simulink model "dspcelpcoder"  (Simulink 6.0)
settings: Solver=FixedStepDiscrete  SolverMode=SingleTasking  StartTime=0.0  StopTime=3  RelTol=1e-3
PreLoadFcn:
  | load lpcvocoder.mat;
values from neighbouring files (symbols this model uses):
  D = var(Noisef)    [lmsxy.m]
  Speech = [0.139446526672 0.138625044925 0.138111618832 0.138471017097 0.138316989269 0.138625044925 0.138419674488 0.137854905786 0.138419674488 0.138111618832 0.138573702316 0.138881757971 ... (24000 elements, 24000x1)]    [lpcvocoder.mat]
undefined symbols (not defined in the file or in its folder): jet, magnitude, poly2lsf
libraries: simulink x25, dspindex x17, dspcelplib x14, dsparch4 x12, dspquant2 x10, dspstat3 x10, dspsrcs4 x8, dspbuff3 x8, dspsigops x7, dspmtrx3 x6, dsplp x5, dspobslib x4
(part 2 of 3)

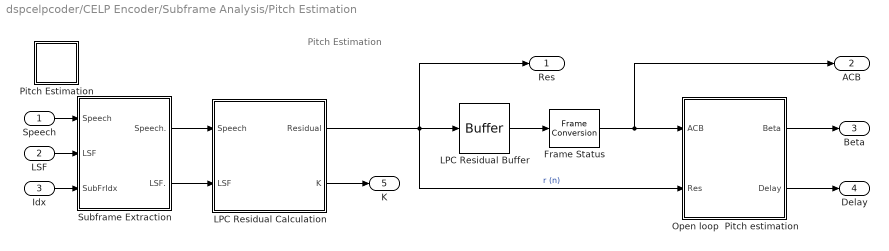
== system dspcelpcoder/CELP Encoder/Subframe Analysis/Pitch Estimation ==
  note: Pitch Estimation
  Speech : Inport  LatchInput=off
  LSF : Inport  Port=2  LatchInput=off
  Idx : Inport  Port=3  LatchInput=off
  Frame Status : FrameConversion  OutFrame=Sample based
  LPC Residual Buffer : dspbuff3/Buffer  N=128+40+20-1  V=187-40  ic=0
  LPC Residual Calculation : Subsystem  PropExecContextAcrossSSBoundary=on
  Open loop  Pitch estimation : Subsystem  PropExecContextAcrossSSBoundary=on
  Pitch Estimation : Subsystem  PropExecContextAcrossSSBoundary=on  mask(DocBlock){ECoderFlag=, DocumentType=Text}
      mask prompts: ECoderFlag "RTW Embedded Coder Flag"; DocumentType "Document Type"
      mask help: Use this block to save long descriptive text with the model. Double-clicking the block will open an editor.
      settings: CopyFcn=docblock('breaklink',gcb);  DeleteFcn=docblock('close_document',gcb);  PreSaveFcn=docblock('save_document',gcb);  OpenFcn=docblock('edit_document',gcb);
      mask StyleString: edit,popup(Text|RTF|HTML)
      mask Display:
      | plot([.8 0 0 1 1 .8 .8 1],[1 1 0 0 .8 1 .8 .8]);
      | text(.5,.5,'DOC','horizontalalignment','center');
  Subframe Extraction : Subsystem  PropExecContextAcrossSSBoundary=on
  Res : Outport
  ACB : Outport  Port=2
  Beta : Outport  Port=3
  Delay : Outport  Port=4
  K : Outport  Port=5
  wires:
  Subframe Extraction/1(Speech.) -> LPC Residual Calculation/1(Speech)
  Subframe Extraction/2(LSF.) -> LPC Residual Calculation/2(LSF)
  LPC Residual Calculation/1(Residual) -> LPC Residual Buffer/1, Open loop  Pitch estimation/2(Res), Res/1  "r (n)"
  LPC Residual Buffer/1 -> Frame Status/1
  Speech/1 -> Subframe Extraction/1(Speech)
  Open loop  Pitch estimation/1(Beta) -> Beta/1
  LSF/1 -> Subframe Extraction/2(LSF)
  LPC Residual Calculation/2(K) -> K/1
  Idx/1 -> Subframe Extraction/3(SubFrIdx)
  Open loop  Pitch estimation/2(Delay) -> Delay/1
  Frame Status/1 -> ACB/1, Open loop  Pitch estimation/1(ACB)

== system dspcelpcoder/CELP Encoder/Subframe Analysis/Pitch Residual computation ==
  note: r (n-D)
  note: beta.r (n-D)
  Res : Inport  LatchInput=off
  ACB : Inport  Port=2  LatchInput=off
  Beta : Inport  Port=3  LatchInput=off
  Delay : Inport  Port=4  LatchInput=off
  Adaptive codebook (ACB) vector candidate  generation : dspcelplib/Select Rows  numRows=40
  DocBlock : Subsystem  PropExecContextAcrossSSBoundary=on  mask(DocBlock){ECoderFlag=, DocumentType=Text}
      mask prompts: ECoderFlag "RTW Embedded Coder Flag"; DocumentType "Document Type"
      mask help: Use this block to save long descriptive text with the model. Double-clicking the block will open an editor.
      settings: CopyFcn=docblock('breaklink',gcb);  DeleteFcn=docblock('close_document',gcb);  PreSaveFcn=docblock('save_document',gcb);  OpenFcn=docblock('edit_document',gcb);
      mask StyleString: edit,popup(Text|RTF|HTML)
      mask Display:
      | plot([.8 0 0 1 1 .8 .8 1],[1 1 0 0 .8 1 .8 .8]);
      | text(.5,.5,'DOC','horizontalalignment','center');
  Frame Status : FrameConversion  OutFrame=Sample based
  Product : Product  SaturateOnIntegerOverflow=on  InputSameDT=on
  SQ (6bits):  Pitch gain (beta) : dspquant2/Scalar Quantizer Encoder  paramSrc=Specify via dialog  partType=Unbounded  BBoundary=[1:10]  UBoundary="[-664.4987     -226.6211     -163.1446     -118.9086     -113.9219     -108.7279     -104.5664     -99.11397     -94.05304     -88.82067     -84.78541     -82.84984      -79.8832     -76.88246     -75.50286     -73.83455     -72.61365     -70.82638      -68.5152     -66.00678     -64.26053     -63.33299     -62.29661     -61.59388     -60.91468      -59.5846     -58.31332     -57.45637     -56.60959     -55.83433     -55.12464     -54.17846     -53.21915     -52.48859     -51.37979     -49.84736     -47.53809     -44.36728     -40.84603     -36.95474     -32.52144     -28.08435     -23.77407     -19.41755     -15.15212     -10.81123      -6.70638     -3.562581     -1.573976    -0.6202197    0.03800587     0.6992125      2.642395      8.360806      18.00463      30.51523      46.10913      64.72121      84.13315       102.069      123.7346      158.1681      206.6721]"  SearchMethod=Binary  tieBreakRule=Choose the lower index  outQU=on  outQError=off  codebook="[-1082.3569     -246.64044     -206.60177     -119.68735     -118.12987     -109.71395     -107.74187     -101.39102     -96.836918     -91.269156     -86.372177     -83.198634     -82.501047     -77.265358     -76.499561     -74.506154     -73.162943     -72.064354     -69.588398     -67.441995     -64.571558     -63.949501     -62.716478     -61.876738     -61.311021     -60.518343     -58.650854     -57.975792     -56.936942     -56.282238     -55.386427     -54.862852     -53.494072      -52.94422     -52.032961      -50.72662     -48.968103      -46.10807       -42.6265     -39.065568     -34.843913     -30.198965     -25.969732     -21.578415     -17.256677     -13.047571     -8.5748944     -4.8378646     -2.2872972    -0.86065481    -0.37978458     0.45579633     0.94262874      4.3421606      12.379451      23.629803       37.40066      54.817595      74.624825      93.641473      110.49643      136.97269      179.36351      233.98073]"  outStatus=off  invalidin=Clip  idtype=int32  roundingMode=Floor  overflowMode=off
  Sum2 : Sum  Inputs=|+-  SaturateOnIntegerOverflow=on
  PitchRes : Outport
  Idx_beta : Outport  Port=2
  wires:
  ACB/1 -> Adaptive codebook (ACB) vector candidate  generation/1
  Sum2/1 -> Frame Status/1
  Res/1 -> Sum2/1  "r(n)"
  Delay/1 -> Adaptive codebook (ACB) vector candidate  generation/2
  Product/1 -> Sum2/2
  Adaptive codebook (ACB) vector candidate  generation/1 -> Product/1
  Beta/1 -> SQ (6bits):  Pitch gain (beta)/1
  SQ (6bits):  Pitch gain (beta)/2 -> Product/2
  SQ (6bits):  Pitch gain (beta)/1 -> Idx_beta/1
  Frame Status/1 -> PitchRes/1

== system dspcelpcoder/CELP Encoder/Subframe Analysis/Subframe Analysis ==
  EmptySubsystem : Subsystem  PropExecContextAcrossSSBoundary=on

== system dspcelpcoder/CELP Decoder/Subframe Synthesis/Formant Post Filter/Subsystem for ARMA Coefficients ==
  Lpc : Inport  LatchInput=off
  Bandwidth Expansion : Subsystem  PropExecContextAcrossSSBoundary=on  mask(Bandwidth Expansion){alpha=0.65}
      mask prompts: alpha "Bandwidth expansion factor:"
      mask help:
      | Generate autoregressive (AR) polynomial with bandwidth expanded relative to the bandwidth of the input AR polynomial.
      |
      | By reducing the radius of the roots in an autoregressive polynomial (i.e., scaling them towards the origin of the Z-plane), the bandwidth of the spectral peaks in the frequency response is expanded (flattened).  This operation is often referred to as "bandwidth expansion".
      |
      | Bandwidth expansion factor must be in the range [0,1], where 1.0 yields no changes to the roots of the polynomial.
      mask Help: web(dspbhelp);
      mask Display: fprintf('Bandwidth\nExpansion\n%g', alpha)
  Bandwidth Expansion1 : Subsystem  PropExecContextAcrossSSBoundary=on  mask(Bandwidth Expansion){alpha=0.75}
      mask prompts: alpha "Bandwidth expansion factor:"
      mask help:
      | Generate autoregressive (AR) polynomial with bandwidth expanded relative to the bandwidth of the input AR polynomial.
      |
      | By reducing the radius of the roots in an autoregressive polynomial (i.e., scaling them towards the origin of the Z-plane), the bandwidth of the spectral peaks in the frequency response is expanded (flattened).  This operation is often referred to as "bandwidth expansion".
      |
      | Bandwidth expansion factor must be in the range [0,1], where 1.0 yields no changes to the roots of the polynomial.
      mask Help: web(dspbhelp);
      mask Display: fprintf('Bandwidth\nExpansion\n%g', alpha)
  FirCoef : Outport
  IirCoef : Outport  Port=2
  wires:
  Lpc/1 -> Bandwidth Expansion/1(In1), Bandwidth Expansion1/1(In1)
  Bandwidth Expansion1/1(Out1) -> IirCoef/1
  Bandwidth Expansion/1(Out1) -> FirCoef/1

== system dspcelpcoder/CELP Decoder/Subframe Synthesis/Gain Scaling Unit/For Iterator Subsystem1 ==
  note: g(n)
  note: y(n)
  note: y(n)=g(n)+0.9375y(n-1)
      | with IC=1
  note: Computation of gain scaling factor for each sample of the subframe
  ScalarGain : Inport  LatchInput=off
  Assignment : Assignment  ElementSrc=External  Rows=-1  ColumnSrc=External
  Constant1 : Constant  Orientation=down  Value=zeros(40,1)  VectorParams1D=off
  For Iterator : ForIterator  IterationLimit=40
  filter : dsparch4/Digital Filter  DialogController=dspDDGCreate  DialogControllerArgs=DataTag8  TypePopup=IIR (all poles)  IIRFiltStruct=Direct form II transposed  AllPoleFiltStruct=Direct form  FIRFiltStruct=Direct form  CoeffSource=Specify via dialog  NumCoeffs=[1 -.95]  DenCoeffs="[1   -0.9375]"  BiQuadCoeffs=[1 0.3 0.4 1 0.1 0.2]  LatticeCoeffs=[0.2 0.4]  denIgnore=on  FiltPerSampPopup=One filter per frame  IC=1  ICnum=0  ICden=0  roundingMode=Floor  overflowMode=off  ScaleValues=1  scaleValueFracLength=14  stageInFracLength=15  stageOutFracLength=15
  VectorGain : Outport
  wires:
  For Iterator/1 -> Assignment/3
  Assignment/1 -> VectorGain/1
  Constant1/1 -> Assignment/1
  ScalarGain/1 -> filter/1
  filter/1 -> Assignment/2

== system dspcelpcoder/CELP Decoder/Subframe Synthesis/Reconstruction of  Speech Subframe/Harmonic Shaper ==
  inRes : Inport  LatchInput=off
  Delay : Inport  Port=2  LatchInput=off
  Beta : Inport  Port=3  LatchInput=off
  1-bz^(-D)2 : Subsystem  TreatAsAtomicUnit=on  PropExecContextAcrossSSBoundary=on
  Energy normalization : Subsystem  PropExecContextAcrossSSBoundary=on
  Pitch Synthesis Filtering 1/(1-b.z^(-D))2 : dsparch4/Digital Filter  DialogController=dspDDGCreate  DialogControllerArgs=DataTag9  TypePopup=IIR (all poles)  IIRFiltStruct=Direct form II transposed  AllPoleFiltStruct=Direct form  FIRFiltStruct=Direct form  CoeffSource=Input port(s)  NumCoeffs=[1 -.95]  DenCoeffs=[1 0.1]  BiQuadCoeffs=[1 0.3 0.4 1 0.1 0.2]  LatticeCoeffs=[0.2 0.4]  denIgnore=on  FiltPerSampPopup=One filter per frame  IC=0  ICnum=0  ICden=0  roundingMode=Floor  overflowMode=off  ScaleValues=1  scaleValueFracLength=14  stageInFracLength=15  stageOutFracLength=15
  OutRes : Outport
  wires:
  Pitch Synthesis Filtering 1/(1-b.z^(-D))2/1 -> Energy normalization/2(SigNew)
  inRes/1 -> Energy normalization/1(SigOrg), Pitch Synthesis Filtering 1/(1-b.z^(-D))2/1
  1-bz^(-D)2/1(Polynom) -> Pitch Synthesis Filtering 1/(1-b.z^(-D))2/2
  Delay/1 -> 1-bz^(-D)2/1(D_buf_1based)
  Beta/1 -> 1-bz^(-D)2/2(beta)
  Energy normalization/1(SigNew2) -> OutRes/1  "res"

== system dspcelpcoder/CELP Decoder/Subframe Synthesis/Reconstruction of  Speech Subframe/LP Synthesis Filter ==
  Residual : Inport  LatchInput=off
  LSF : Inport  Port=2  LatchInput=off
  LPC to/from RC : dsplp/LPC to//from RC  conversion=LPC to RC  perr=off  stability=off  error=Replace it with 1
  LSF/LSP to LPC Conversion : dsplp/LSF//LSP to LPC Conversion  input=LSF in range (0 pi)
  Time-Varying  Synthesis Filter 1/A(z) : dsparch4/Digital Filter  DialogController=dspDDGCreate  DialogControllerArgs=DataTag10  TypePopup=IIR (all poles)  IIRFiltStruct=Direct form II transposed  AllPoleFiltStruct=Lattice AR  FIRFiltStruct=Direct form  CoeffSource=Input port(s)  NumCoeffs=[1 -.95]  DenCoeffs=[1 0.1]  BiQuadCoeffs=[1 0.3 0.4 1 0.1 0.2]  LatticeCoeffs=[0.2 0.4]  denIgnore=off  FiltPerSampPopup=One filter per frame  IC=0  ICnum=0  ICden=0  roundingMode=Floor  overflowMode=off  ScaleValues=1  scaleValueFracLength=14  stageInFracLength=15  stageOutFracLength=15
  Sig : Outport
  LPC : Outport  Port=2
  wires:
  LSF/LSP to LPC Conversion/1 -> LPC to/from RC/1, LPC/1
  LPC to/from RC/1 -> Time-Varying  Synthesis Filter 1/A(z)/2
  Residual/1 -> Time-Varying  Synthesis Filter 1/A(z)/1
  Time-Varying  Synthesis Filter 1/A(z)/1 -> Sig/1  "S(n)"
  LSF/1 -> LSF/LSP to LPC Conversion/1

== system dspcelpcoder/CELP Decoder/Subframe Synthesis/Reconstruction of  Speech Subframe/Pitch synthesis ==
  PitchRes : Inport  LatchInput=off
  Delay : Inport  Port=2  LatchInput=off
  Beta : Inport  Port=3  LatchInput=off
  1-bz^(-D) : Subsystem  TreatAsAtomicUnit=on  PropExecContextAcrossSSBoundary=on
  Pitch synthesis Filter 1/(1-b.z^(-D)) : dsparch4/Digital Filter  DialogController=dspDDGCreate  DialogControllerArgs=DataTag11  TypePopup=IIR (all poles)  IIRFiltStruct=Direct form II transposed  AllPoleFiltStruct=Direct form  FIRFiltStruct=Direct form  CoeffSource=Input port(s)  NumCoeffs=[1 -.95]  DenCoeffs=[1 0.1]  BiQuadCoeffs=[1 0.3 0.4 1 0.1 0.2]  LatticeCoeffs=[0.2 0.4]  denIgnore=on  FiltPerSampPopup=One filter per frame  IC=0  ICnum=0  ICden=0  roundingMode=Floor  overflowMode=off  ScaleValues=1  scaleValueFracLength=14  stageInFracLength=15  stageOutFracLength=15
  LPRes : Outport
  wires:
  1-bz^(-D)/1(Polynom) -> Pitch synthesis Filter 1/(1-b.z^(-D))/2
  Delay/1 -> 1-bz^(-D)/1(D_buf_1based)
  Beta/1 -> 1-bz^(-D)/2(beta)
  PitchRes/1 -> Pitch synthesis Filter 1/(1-b.z^(-D))/1
  Pitch synthesis Filter 1/(1-b.z^(-D))/1 -> LPRes/1

== system dspcelpcoder/CELP Decoder/Subframe Synthesis/Reconstruction of  Speech Subframe/Reconstruction of  Pitch Residual Signal ==
  4SignBit : Inport  LatchInput=off
  4Position : Inport  Port=2  LatchInput=off
  FCBgain : Inport  Port=3  LatchInput=off
  Frame Status : FrameConversion  OutFrame=Sample based
  Frame Status1 : FrameConversion  OutFrame=Sample based
  Product4 : Product  OutDataTypeMode=double  SaturateOnIntegerOverflow=on
  replace 4 selected samples by their sign and set others to zero : Subsystem  TreatAsAtomicUnit=on  PropExecContextAcrossSSBoundary=on
  qPitchRes : Outport
  wires:
  Frame Status/1 -> replace 4 selected samples by their sign and set others to zero/1(4SignBit)
  Frame Status1/1 -> replace 4 selected samples by their sign and set others to zero/2(4Position)
  replace 4 selected samples by their sign and set others to zero/1(newPitchRes) -> Product4/1
  4SignBit/1 -> Frame Status/1
  4Position/1 -> Frame Status1/1
  Product4/1 -> qPitchRes/1
  FCBgain/1 -> Product4/2

== system dspcelpcoder/CELP Encoder/Frame Analysis/Classical LPC analysis/Bandwidth Expansion ==
  In1 : Inport  LatchInput=off
  Window Function : dspsigops/Window Function  DialogController=dspDDGCreate  DialogControllerArgs=DataTag14  winmode=Apply window to input  wintype=User defined  sampmode=Continuous  samptime=1  N=64  Rs=50  beta=10  winsamp=Symmetric  UserWindow=bwexpwin  OptParams=on  UserParams=alpha  dataType=double  isSigned=on  wordLen=16  udDataType=sfix(16)  fracBitsMode=Best precision  numFracBits=15  roundingMode=Floor  overflowMode=off
  Out1 : Outport
  wires:
  In1/1 -> Window Function/1
  Window Function/1 -> Out1/1

== system dspcelpcoder/CELP Encoder/Frame Analysis/Classical LPC analysis/LPC Analysis ==
  EmptySubsystem : Subsystem  PropExecContextAcrossSSBoundary=on

== system dspcelpcoder/CELP Encoder/Frame Analysis/LSF Interpolation/LSF Interpolation ==
  EmptySubsystem : Subsystem  PropExecContextAcrossSSBoundary=on

== system dspcelpcoder/CELP Encoder/Frame Analysis/LSF Vector Quantization/LSF Split VQ ==
  EmptySubsystem : Subsystem  PropExecContextAcrossSSBoundary=on

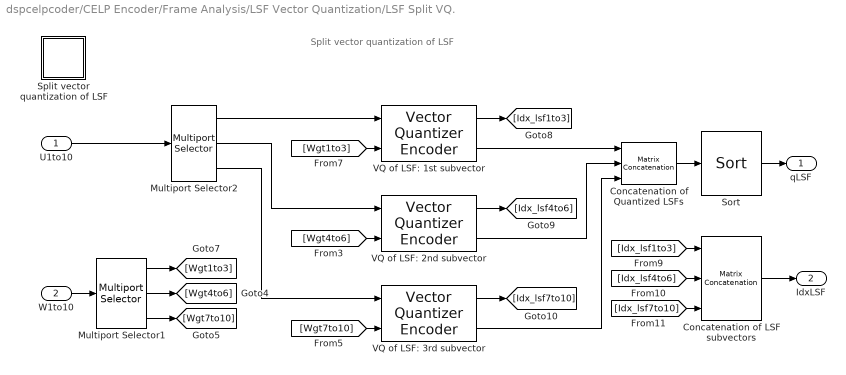
== system dspcelpcoder/CELP Encoder/Frame Analysis/LSF Vector Quantization/LSF Split VQ. ==
  note: Split vector quantization of LSF
  U1to10 : Inport  LatchInput=off
  W1to10 : Inport  Port=2  LatchInput=off
  Concatenation of LSF subvectors : simulink/Math Operations/Matrix Concatenation  numInports=3  catMethod=Horizontal
  Concatenation of Quantized LSFs : simulink/Math Operations/Matrix Concatenation  numInports=3  catMethod=Vertical
  Multiport Selector1 : dspindex/Multiport Selector  rowsOrCols=Rows  idxCellArray={1:3,4:6,7:10}  idxErrMode=Clip Index
  Multiport Selector2 : dspindex/Multiport Selector  rowsOrCols=Rows  idxCellArray={1:3,4:6,7:10}  idxErrMode=Clip Index
  Sort : dspstat3/Sort  DialogController=dspDDGCreate  DialogControllerArgs=DataTag17  otype=Value  dir=Ascending  sortAlg=Quick sort  roundingMode=Floor  overflowMode=off
  Split vector quantization of LSF : Subsystem  PropExecContextAcrossSSBoundary=on  mask(DocBlock){ECoderFlag=, DocumentType=Text}
      mask prompts: ECoderFlag "RTW Embedded Coder Flag"; DocumentType "Document Type"
      mask help: Use this block to save long descriptive text with the model. Double-clicking the block will open an editor.
      settings: CopyFcn=docblock('breaklink',gcb);  DeleteFcn=docblock('close_document',gcb);  PreSaveFcn=docblock('save_document',gcb);  OpenFcn=docblock('edit_document',gcb);
      mask StyleString: edit,popup(Text|RTF|HTML)
      mask Display:
      | plot([.8 0 0 1 1 .8 .8 1],[1 1 0 0 .8 1 .8 .8]);
      | text(.5,.5,'DOC','horizontalalignment','center');
  VQ of LSF: 1st subvector : dspquant2/Vector Quantizer Encoder  CBsource=Specify via dialog  codebook=CB_lsf1to3_10bit  distMeasure=Weighted squared error  wgtSrc=Input port  weights=[1 1 1]  tieBreakRule=Choose the lower index  outQU=on  outQError=off  idtype=int32  roundingMode=Floor  overflowMode=off
  VQ of LSF: 2nd subvector : dspquant2/Vector Quantizer Encoder  CBsource=Specify via dialog  codebook=CB_lsf4to6_10bit  distMeasure=Weighted squared error  wgtSrc=Input port  weights=[1 1 1]  tieBreakRule=Choose the lower index  outQU=on  outQError=off  idtype=int32  roundingMode=Floor  overflowMode=off
  VQ of LSF: 3rd subvector : dspquant2/Vector Quantizer Encoder  CBsource=Specify via dialog  codebook=CB_lsf7to10_10bit  distMeasure=Weighted squared error  wgtSrc=Input port  weights=[1 1 1]  tieBreakRule=Choose the lower index  outQU=on  outQError=off  idtype=int32  roundingMode=Floor  overflowMode=off
  qLSF : Outport
  IdxLSF : Outport  Port=2
  wires:
  VQ of LSF: 1st subvector/2 -> Concatenation of Quantized LSFs/1
  VQ of LSF: 1st subvector/1 -> [Idx_lsf1to3]
  Multiport Selector2/2 -> VQ of LSF: 2nd subvector/1
  Multiport Selector2/3 -> VQ of LSF: 3rd subvector/1
  Multiport Selector1/2 -> [Wgt4to6]
  Multiport Selector1/3 -> [Wgt7to10]
  VQ of LSF: 2nd subvector/1 -> [Idx_lsf4to6]
  [Wgt7to10] -> VQ of LSF: 3rd subvector/2
  VQ of LSF: 3rd subvector/1 -> [Idx_lsf7to10]
  VQ of LSF: 2nd subvector/2 -> Concatenation of Quantized LSFs/2
  Concatenation of Quantized LSFs/1 -> Sort/1
  VQ of LSF: 3rd subvector/2 -> Concatenation of Quantized LSFs/3
  [Wgt4to6] -> VQ of LSF: 2nd subvector/2
  Multiport Selector1/1 -> [Wgt1to3]
  [Wgt1to3] -> VQ of LSF: 1st subvector/2
  [Idx_lsf1to3] -> Concatenation of LSF subvectors/1
  [Idx_lsf4to6] -> Concatenation of LSF subvectors/2
  [Idx_lsf7to10] -> Concatenation of LSF subvectors/3
  W1to10/1 -> Multiport Selector1/1
  U1to10/1 -> Multiport Selector2/1
  Sort/1 -> qLSF/1
  Concatenation of LSF subvectors/1 -> IdxLSF/1
  Multiport Selector2/1 -> VQ of LSF: 1st subvector/1

== system dspcelpcoder/CELP Encoder/Frame Analysis/LSF Vector Quantization/Paliwal Weight  Computation ==
  note: Calculation of Perceptual Weighting Factors
  LSF : Inport  LatchInput=off
  LPC : Inport  Port=2  LatchInput=off
  Calculation of Perceptual  Weighting Factors : Subsystem  PropExecContextAcrossSSBoundary=on  mask(DocBlock){ECoderFlag=, DocumentType=Text}
      mask prompts: ECoderFlag "RTW Embedded Coder Flag"; DocumentType "Document Type"
      mask help: Use this block to save long descriptive text with the model. Double-clicking the block will open an editor.
      settings: CopyFcn=docblock('breaklink',gcb);  DeleteFcn=docblock('close_document',gcb);  PreSaveFcn=docblock('save_document',gcb);  OpenFcn=docblock('edit_document',gcb);
      mask StyleString: edit,popup(Text|RTF|HTML)
      mask Display:
      | plot([.8 0 0 1 1 .8 .8 1],[1 1 0 0 .8 1 .8 .8]);
      | text(.5,.5,'DOC','horizontalalignment','center');
  Constant : Constant  Orientation=up  Value=0.15  VectorParams1D=off  SampleTime=-1
  DSP Gain2 : dspobslib/DSP Gain  gainValue=[ones(1,8) 0.8 0.4]  roundingMode=Floor  overflowMode=off
  DSP Gain3 : dspobslib/DSP Gain  gainValue=-1  roundingMode=Floor  overflowMode=off
  LPCpowSpec : Subsystem  PropExecContextAcrossSSBoundary=on
  Math Function : Math  Operator=pow  SaturateOnIntegerOverflow=on
  Reshape : simulink/Math Operations/Reshape  OutputDimensionality=Column vector  OutputDimensions=[1,1]
  Submatrix : dspmtrx3/Submatrix  RowSpan=Range of rows  RowStartMode=Index  RowStartIndex=2  RowEndMode=Last  RowEndIndex=1  ColSpan=All columns  ColStartMode=First  ColStartIndex=1  ColEndMode=Last  ColEndIndex=1
  Weights : Outport
  wires:
  LPCpowSpec/1(Out) -> Math Function/1
  Constant/1 -> Math Function/2
  Math Function/1 -> DSP Gain2/1
  DSP Gain2/1 -> Reshape/1
  LSF/1 -> LPCpowSpec/2(LSF)
  Reshape/1 -> Weights/1
  Submatrix/1 -> DSP Gain3/1
  LPC/1 -> Submatrix/1
  DSP Gain3/1 -> LPCpowSpec/1(PC)

== system dspcelpcoder/CELP Encoder/Frame Analysis/Subframe Analysis/EmptySubsystem ==

== system dspcelpcoder/CELP Encoder/Subframe Analysis/Innovation signal quantization/DocBlock ==
  EmptySubsystem : Subsystem  PropExecContextAcrossSSBoundary=on

== system dspcelpcoder/CELP Encoder/Subframe Analysis/Innovation signal quantization/Impulse Response ==
  In1 : Inport  LatchInput=off
  DSP Constant : dspsrcs4/DSP Constant  Value=[1;zeros(39,1)]  SampleMode=Discrete  discreteOutput=Frame-based  continuousOutput=Sample-based  sampTime=1  framePeriod=-1  dataType=Inherit from 'Constant value'  isSigned=on  wordLen=16  udDataType=sfix(16)  fracBitsMode=Best precision  numFracBits=15  InterpretAs1D=-inf  Ts=-inf  FramebasedOutput=-inf
  For Iterator Subsystem2 : Subsystem  TreatAsAtomicUnit=on  PropExecContextAcrossSSBoundary=on
      mask Display:
      | disp('Zero State\nIIR Lattice\nFilter');
      | port_label('input',1,'In');
      | port_label('input',2,'K');
      | port_label('output',1,'Out');
  Out1 : Outport
  wires:
  For Iterator Subsystem2/1(SigOut2) -> Out1/1
  In1/1 -> For Iterator Subsystem2/2(K)
  DSP Constant/1 -> For Iterator Subsystem2/1(SigIn2)

== system dspcelpcoder/CELP Encoder/Subframe Analysis/Innovation signal quantization/Searching for FCB pulse  positions and FCB gain ==
  note: To Search for FCB pulse positions and FCB gain
  PitchRes : Inport  LatchInput=off
  Idx : Inport  Port=2  LatchInput=off
  e_n : Inport  Port=3  LatchInput=off
  h : Inport  Port=4  LatchInput=off
  1-based to  0-based : Bias  Bias=-1
  Computation of  Error and Gain : Subsystem  PropExecContextAcrossSSBoundary=on
  For Iterator : ForIterator  ResetStates=reset  IterationLimit=37
  Optimal Features : Subsystem  PropExecContextAcrossSSBoundary=on
  Partial decomposition of  Pitch Residual : Subsystem  PropExecContextAcrossSSBoundary=on
  Searching for FCB features : Subsystem  PropExecContextAcrossSSBoundary=on  mask(DocBlock){ECoderFlag=, DocumentType=Text}
      mask prompts: ECoderFlag "RTW Embedded Coder Flag"; DocumentType "Document Type"
      mask help: Use this block to save long descriptive text with the model. Double-clicking the block will open an editor.
      settings: CopyFcn=docblock('breaklink',gcb);  DeleteFcn=docblock('close_document',gcb);  PreSaveFcn=docblock('save_document',gcb);  OpenFcn=docblock('edit_document',gcb);
      mask StyleString: edit,popup(Text|RTF|HTML)
      mask Display:
      | plot([.8 0 0 1 1 .8 .8 1],[1 1 0 0 .8 1 .8 .8]);
      | text(.5,.5,'DOC','horizontalalignment','center');
  Signal to sign bit : Subsystem  PropExecContextAcrossSSBoundary=on
  pos_sign_g : Outport
  wires:
  1-based to  0-based/1 -> Computation of  Error and Gain/2(4Pos)
  h/1 -> Computation of  Error and Gain/4(h)
  e_n/1 -> Computation of  Error and Gain/3(e_n)
  Signal to sign bit/1(SignBit) -> Computation of  Error and Gain/1(4Val), Optimal Features/1(SignBit)
  Partial decomposition of  Pitch Residual/2(4Idx) -> 1-based to  0-based/1, Optimal Features/4(Pos)
  Partial decomposition of  Pitch Residual/1(4Val) -> Signal to sign bit/1(Sig)
  For Iterator/1 -> Partial decomposition of  Pitch Residual/3(Control)
  Idx/1 -> Partial decomposition of  Pitch Residual/2(Idx)
  PitchRes/1 -> Partial decomposition of  Pitch Residual/1(PitchRes)
  Computation of  Error and Gain/1(Err) -> Optimal Features/2(Err)
  Computation of  Error and Gain/2(G) -> Optimal Features/3(G)
  Optimal Features/1(Features) -> pos_sign_g/1

== system dspcelpcoder/CELP Encoder/Subframe Analysis/Innovation signal quantization/filter ==
  SigIn2 : Inport  LatchInput=off
  K : Inport  Port=2  LatchInput=off
  DocBlock : Subsystem  PropExecContextAcrossSSBoundary=on  mask(DocBlock){ECoderFlag=, DocumentType=Text}
      mask prompts: ECoderFlag "RTW Embedded Coder Flag"; DocumentType "Document Type"
      mask help: Use this block to save long descriptive text with the model. Double-clicking the block will open an editor.
      settings: CopyFcn=docblock('breaklink',gcb);  DeleteFcn=docblock('close_document',gcb);  PreSaveFcn=docblock('save_document',gcb);  OpenFcn=docblock('edit_document',gcb);
      mask StyleString: edit,popup(Text|RTF|HTML)
      mask Display:
      | plot([.8 0 0 1 1 .8 .8 1],[1 1 0 0 .8 1 .8 .8]);
      | text(.5,.5,'DOC','horizontalalignment','center');
  For Iterator : ForIterator  ResetStates=reset  IterationLimit=1  ShowIterationPort=off
  Time-Varying  Synthesis Filter 1/A(z). : dsparch4/Digital Filter  DialogController=dspDDGCreate  DialogControllerArgs=DataTag22  TypePopup=IIR (all poles)  IIRFiltStruct=Direct form II transposed  AllPoleFiltStruct=Lattice AR  FIRFiltStruct=Direct form  CoeffSource=Input port(s)  NumCoeffs=[1 -.95]  DenCoeffs=[1 0.1]  BiQuadCoeffs=[1 0.3 0.4 1 0.1 0.2]  LatticeCoeffs=[0.2 0.4]  denIgnore=off  FiltPerSampPopup=One filter per frame  IC=0  ICnum=0  ICden=0  roundingMode=Floor  overflowMode=off  ScaleValues=1  scaleValueFracLength=14  stageInFracLength=15  stageOutFracLength=15
  SigOut2 : Outport
  wires:
  Time-Varying  Synthesis Filter 1/A(z)./1 -> SigOut2/1
  SigIn2/1 -> Time-Varying  Synthesis Filter 1/A(z)./1
  K/1 -> Time-Varying  Synthesis Filter 1/A(z)./2

== system dspcelpcoder/CELP Encoder/Subframe Analysis/Pitch Estimation/LPC Residual Calculation ==
  Speech : Inport  LatchInput=off
  LSF : Inport  Port=2  LatchInput=off
  LPC to/from RC : dsplp/LPC to//from RC  conversion=LPC to RC  perr=off  stability=off  error=Replace it with 1
  LSF/LSP to LPC Conversion : dsplp/LSF//LSP to LPC Conversion  input=LSF in range (0 pi)
  Time-Varying  Analysis Filter A(z) : dsparch4/Digital Filter  DialogController=dspDDGCreate  DialogControllerArgs=DataTag23  TypePopup=FIR (all zeros)  IIRFiltStruct=Direct form II transposed  AllPoleFiltStruct=Direct form  FIRFiltStruct=Lattice MA  CoeffSource=Input port(s)  NumCoeffs=[1 -.95]  DenCoeffs=[1 0.1]  BiQuadCoeffs=[1 0.3 0.4 1 0.1 0.2]  LatticeCoeffs=[0.2 0.4]  denIgnore=on  FiltPerSampPopup=One filter per frame  IC=0  ICnum=0  ICden=0  roundingMode=Floor  overflowMode=off  ScaleValues=1  scaleValueFracLength=14  stageInFracLength=15  stageOutFracLength=15
  Residual : Outport
  K : Outport  Port=2
  wires:
  LSF/LSP to LPC Conversion/1 -> LPC to/from RC/1
  Speech/1 -> Time-Varying  Analysis Filter A(z)/1
  Time-Varying  Analysis Filter A(z)/1 -> Residual/1
  LSF/1 -> LSF/LSP to LPC Conversion/1
  LPC to/from RC/1 -> Time-Varying  Analysis Filter A(z)/2, K/1

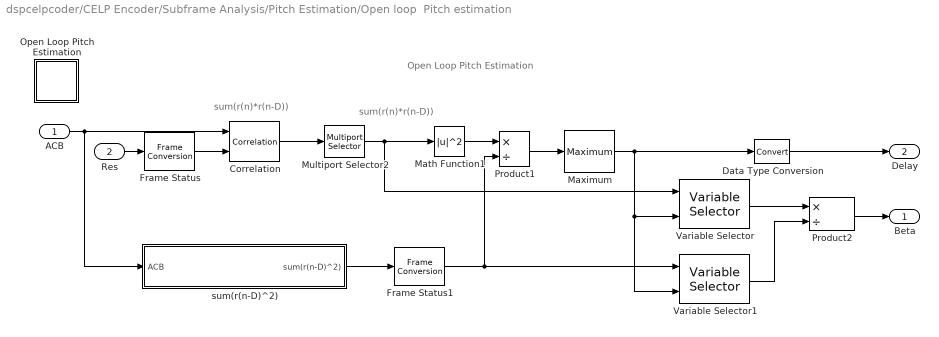
== system dspcelpcoder/CELP Encoder/Subframe Analysis/Pitch Estimation/Open loop  Pitch estimation ==
  note: sum(r(n)*r(n-D))
  note: sum(r(n)*r(n-D))
  note: Open Loop Pitch Estimation
  ACB : Inport  LatchInput=off
  Res : Inport  Port=2  LatchInput=off
  Correlation : dspstat3/Correlation  DialogController=dspDDGCreate  DialogControllerArgs=DataTag24  domain=Fastest  roundingMode=Floor  overflowMode=off
  Data Type Conversion : DataTypeConversion  OutDataTypeMode=int32  SaturateOnIntegerOverflow=on  RndMeth=Zero
  Frame Status : FrameConversion  OutFrame=Sample based
  Frame Status1 : FrameConversion  OutFrame=Sample based
  Math Function1 : Math  Operator=magnitude^2  SaturateOnIntegerOverflow=on
  Maximum : dspstat3/Maximum  DialogController=dspDDGCreate  DialogControllerArgs=DataTag25  fcn=Index  reset=None  roundingMode=Floor  overflowMode=off
  Multiport Selector2 : dspindex/Multiport Selector  rowsOrCols=Rows  idxCellArray={40:167}  idxErrMode=Clip Index
  Open Loop Pitch Estimation : Subsystem  PropExecContextAcrossSSBoundary=on  mask(DocBlock){ECoderFlag=, DocumentType=Text}
      mask prompts: ECoderFlag "RTW Embedded Coder Flag"; DocumentType "Document Type"
      mask help: Use this block to save long descriptive text with the model. Double-clicking the block will open an editor.
      settings: CopyFcn=docblock('breaklink',gcb);  DeleteFcn=docblock('close_document',gcb);  PreSaveFcn=docblock('save_document',gcb);  OpenFcn=docblock('edit_document',gcb);
      mask StyleString: edit,popup(Text|RTF|HTML)
      mask Display:
      | plot([.8 0 0 1 1 .8 .8 1],[1 1 0 0 .8 1 .8 .8]);
      | text(.5,.5,'DOC','horizontalalignment','center');
  Product1 : Product  Inputs=*/  SaturateOnIntegerOverflow=on
  Product2 : Product  Inputs=*/  SaturateOnIntegerOverflow=on
  Variable Selector : dspindex/Variable Selector  rowsOrCols=Rows  IdxMode=Variable  Elements=[1 3]  ZerOneIdxMode=One-based  errmode=Generate Error
  Variable Selector1 : dspindex/Variable Selector  rowsOrCols=Rows  IdxMode=Variable  Elements=[1 3]  ZerOneIdxMode=One-based  errmode=Generate Error
  sum(r(n-D)^2) : Subsystem  TreatAsAtomicUnit=on  PropExecContextAcrossSSBoundary=on
  Beta : Outport
  Delay : Outport  Port=2
  wires:
  Product2/1 -> Beta/1
  Variable Selector/1 -> Product2/1
  Maximum/1 -> Variable Selector1/2, Variable Selector/2, Data Type Conversion/1
  Product1/1 -> Maximum/1
  sum(r(n-D)^2)/1(sum(r(n-D)^2)) -> Frame Status1/1
  Math Function1/1 -> Product1/1
  Res/1 -> Frame Status/1
  ACB/1 -> Correlation/1, sum(r(n-D)^2)/1(ACB)
  Multiport Selector2/1 -> Variable Selector/1, Math Function1/1
  Correlation/1 -> Multiport Selector2/1
  Variable Selector1/1 -> Product2/2
  Frame Status/1 -> Correlation/2
  Frame Status1/1 -> Variable Selector1/1, Product1/2
  Data Type Conversion/1 -> Delay/1

== system dspcelpcoder/CELP Encoder/Subframe Analysis/Pitch Estimation/Pitch Estimation ==
  EmptySubsystem : Subsystem  PropExecContextAcrossSSBoundary=on

== system dspcelpcoder/CELP Encoder/Subframe Analysis/Pitch Estimation/Subframe Extraction ==
  Speech : Inport  LatchInput=off
  LSF : Inport  Port=2  LatchInput=off
  SubFrIdx : Inport  Orientation=up  Port=3  LatchInput=off
  Frame to subframe : simulink/Math Operations/Reshape  OutputDimensionality=Customize  OutputDimensions=[40,4]
  Variable Selector : dspindex/Variable Selector  rowsOrCols=Columns  IdxMode=Variable  Elements=[1 3]  ZerOneIdxMode=One-based  errmode=Generate Error
  Variable Selector2 : dspindex/Variable Selector  rowsOrCols=Columns  IdxMode=Variable  Elements=[1 3]  ZerOneIdxMode=One-based  errmode=Generate Error
  Speech. : Outport
  LSF. : Outport  Port=2
  wires:
  SubFrIdx/1 -> Variable Selector/2, Variable Selector2/2
  Speech/1 -> Frame to subframe/1
  Variable Selector/1 -> Speech./1
  LSF/1 -> Variable Selector2/1
  Variable Selector2/1 -> LSF./1
  Frame to subframe/1 -> Variable Selector/1

== system dspcelpcoder/CELP Encoder/Subframe Analysis/Pitch Residual computation/DocBlock ==
  EmptySubsystem : Subsystem  PropExecContextAcrossSSBoundary=on

== system dspcelpcoder/CELP Encoder/Subframe Analysis/Subframe Analysis/EmptySubsystem ==

== system dspcelpcoder/CELP Decoder/Subframe Synthesis/Formant Post Filter/Subsystem for ARMA Coefficients/Bandwidth Expansion ==
  In1 : Inport  LatchInput=off
  Window Function : dspsigops/Window Function  DialogController=dspDDGCreate  DialogControllerArgs=DataTag4  winmode=Apply window to input  wintype=User defined  sampmode=Continuous  samptime=1  N=64  Rs=50  beta=10  winsamp=Symmetric  UserWindow=bwexpwin  OptParams=on  UserParams=alpha  dataType=double  isSigned=on  wordLen=16  udDataType=sfix(16)  fracBitsMode=Best precision  numFracBits=15  roundingMode=Floor  overflowMode=off
  Out1 : Outport
  wires:
  Window Function/1 -> Out1/1
  In1/1 -> Window Function/1

== system dspcelpcoder/CELP Decoder/Subframe Synthesis/Formant Post Filter/Subsystem for ARMA Coefficients/Bandwidth Expansion1 ==
  In1 : Inport  LatchInput=off
  Window Function : dspsigops/Window Function  DialogController=dspDDGCreate  DialogControllerArgs=DataTag5  winmode=Apply window to input  wintype=User defined  sampmode=Continuous  samptime=1  N=64  Rs=50  beta=10  winsamp=Symmetric  UserWindow=bwexpwin  OptParams=on  UserParams=alpha  dataType=double  isSigned=on  wordLen=16  udDataType=sfix(16)  fracBitsMode=Best precision  numFracBits=15  roundingMode=Floor  overflowMode=off
  Out1 : Outport
  wires:
  In1/1 -> Window Function/1
  Window Function/1 -> Out1/1

== system dspcelpcoder/CELP Decoder/Subframe Synthesis/Reconstruction of  Speech Subframe/Harmonic Shaper/1-bz^(-D)2 ==
  note: 187-40+2 = 149
  D_buf_1based : Inport  LatchInput=off
  beta : Inport  Port=2  LatchInput=off
  Assignment1 : Assignment  ElementSrc=External  Rows=-1  ColumnSrc=External
  DSP Constant : dspsrcs4/DSP Constant  Value=[1 zeros(1,187)]'  SampleMode=Discrete  discreteOutput=Frame-based  continuousOutput=Sample-based  sampTime=1  framePeriod=-1  dataType=double  isSigned=on  wordLen=16  udDataType=sfix(16)  fracBitsMode=Best precision  numFracBits=15  InterpretAs1D=-inf  Ts=-inf  FramebasedOutput=-inf
      settings: additionalParams=on
  DSP Constant1 : dspsrcs4/DSP Constant  Orientation=up  Value=149  SampleMode=Discrete  discreteOutput=Frame-based  continuousOutput=Sample-based  sampTime=-1  framePeriod=-1  dataType=Inherit from 'Constant value'  isSigned=on  wordLen=16  udDataType=sfix(16)  fracBitsMode=Best precision  numFracBits=15  InterpretAs1D=-inf  Ts=-inf  FramebasedOutput=-inf
  DSP Gain : dspobslib/DSP Gain  gainValue=-0.965  roundingMode=Floor  overflowMode=off
  For Iterator : ForIterator  ResetStates=reset  IterationLimit=1  ShowIterationPort=off
  Frame Status1 : FrameConversion  OutFrame=Sample based
  Frame Status2 : FrameConversion  OutFrame=Sample based
  Sum3 : Sum  Inputs=|-+  SaturateOnIntegerOverflow=on
  Polynom : Outport
  wires:
  D_buf_1based/1 -> Sum3/1
  Frame Status2/1 -> Assignment1/3
  DSP Gain/1 -> Assignment1/2
  Sum3/1 -> Frame Status2/1
  DSP Constant1/1 -> Sum3/2
  Frame Status1/1 -> DSP Gain/1
  Assignment1/1 -> Polynom/1
  DSP Constant/1 -> Assignment1/1
  beta/1 -> Frame Status1/1

== system dspcelpcoder/CELP Decoder/Subframe Synthesis/Reconstruction of  Speech Subframe/Harmonic Shaper/Energy normalization ==
  SigOrg : Inport  LatchInput=off
  SigNew : Inport  Port=2  LatchInput=off
  DSP Constant : dspsrcs4/DSP Constant  Orientation=up  Value=eps  SampleMode=Discrete  discreteOutput=Frame-based  continuousOutput=Sample-based  sampTime=1  framePeriod=-1  dataType=Inherit from 'Constant value'  isSigned=on  wordLen=16  udDataType=sfix(16)  fracBitsMode=Best precision  numFracBits=15  InterpretAs1D=-inf  Ts=-inf  FramebasedOutput=-inf
  Math Function1 : Math  Operator=sqrt  SaturateOnIntegerOverflow=on
  Product1 : Product  Inputs=*/  SaturateOnIntegerOverflow=on
  Product2 : Product  SaturateOnIntegerOverflow=on
  Subsystem1 : Subsystem  PropExecContextAcrossSSBoundary=on
      mask Display: disp('Energy\nCalculation')
  Subsystem2 : Subsystem  PropExecContextAcrossSSBoundary=on
      mask Display: disp('Energy\nCalculation')
  Sum3 : Sum  Inputs=|++  SaturateOnIntegerOverflow=on
  SigNew2 : Outport
  wires:
  Product2/1 -> SigNew2/1
  SigOrg/1 -> Subsystem1/1(In1)
  SigNew/1 -> Product2/2, Subsystem2/1(In1)
  Math Function1/1 -> Product2/1
  Product1/1 -> Math Function1/1
  Subsystem1/1(Out1) -> Product1/1
  Sum3/1 -> Product1/2
  Subsystem2/1(Out1) -> Sum3/1
  DSP Constant/1 -> Sum3/2

== system dspcelpcoder/CELP Decoder/Subframe Synthesis/Reconstruction of  Speech Subframe/Pitch synthesis/1-bz^(-D) ==
  D_buf_1based : Inport  LatchInput=off
  beta : Inport  Port=2  LatchInput=off
  Assignment1 : Assignment  ElementSrc=External  Rows=-1  ColumnSrc=External
  DSP Constant : dspsrcs4/DSP Constant  Value=[1 zeros(1,187)]'  SampleMode=Discrete  discreteOutput=Frame-based  continuousOutput=Sample-based  sampTime=1  framePeriod=-1  dataType=double  isSigned=on  wordLen=16  udDataType=sfix(16)  fracBitsMode=Best precision  numFracBits=15  InterpretAs1D=-inf  Ts=-inf  FramebasedOutput=-inf
      settings: additionalParams=on
  DSP Constant1 : dspsrcs4/DSP Constant  Orientation=up  Value=149  SampleMode=Discrete  discreteOutput=Frame-based  continuousOutput=Sample-based  sampTime=-1  framePeriod=-1  dataType=int32  isSigned=on  wordLen=16  udDataType=sfix(16)  fracBitsMode=Best precision  numFracBits=15  InterpretAs1D=-inf  Ts=-inf  FramebasedOutput=-inf
      settings: additionalParams=on
  DSP Gain : dspobslib/DSP Gain  gainValue=-1  roundingMode=Floor  overflowMode=off
  For Iterator : ForIterator  ResetStates=reset  IterationLimit=1  ShowIterationPort=off
  Frame Status : FrameConversion  OutFrame=Sample based
  Frame Status1 : FrameConversion  OutFrame=Sample based
  Sum3 : Sum  Inputs=|-+  SaturateOnIntegerOverflow=on
  Polynom : Outport
  wires:
  beta/1 -> Frame Status1/1
  DSP Constant/1 -> Assignment1/1
  Assignment1/1 -> Polynom/1
  Frame Status1/1 -> DSP Gain/1
  DSP Constant1/1 -> Sum3/2
  Sum3/1 -> Frame Status/1
  DSP Gain/1 -> Assignment1/2
  Frame Status/1 -> Assignment1/3
  D_buf_1based/1 -> Sum3/1

== system dspcelpcoder/CELP Decoder/Subframe Synthesis/Reconstruction of  Speech Subframe/Reconstruction of  Pitch Residual Signal/replace 4 selected samples by their sign and set others to zero ==
  4SignBit : Inport  LatchInput=off
  4Position : Inport  Port=2  LatchInput=off
  DocBlock : Subsystem  PropExecContextAcrossSSBoundary=on  mask(DocBlock){ECoderFlag=, DocumentType=Text}
      mask prompts: ECoderFlag "RTW Embedded Coder Flag"; DocumentType "Document Type"
      mask help: Use this block to save long descriptive text with the model. Double-clicking the block will open an editor.
      settings: CopyFcn=docblock('breaklink',gcb);  DeleteFcn=docblock('close_document',gcb);  PreSaveFcn=docblock('save_document',gcb);  OpenFcn=docblock('edit_document',gcb);
      mask StyleString: edit,popup(Text|RTF|HTML)
      mask Display:
      | plot([.8 0 0 1 1 .8 .8 1],[1 1 0 0 .8 1 .8 .8]);
      | text(.5,.5,'DOC','horizontalalignment','center');
  For Iterator : ForIterator  ResetStates=reset  IterationLimit=1  ShowIterationPort=off
  Log all channels1 : dspcelplib/Log all channels  outType=Column vector  numRow=40  numCol=4  dType=int32
  newPitchRes : Outport
  wires:
  4SignBit/1 -> Log all channels1/1
  4Position/1 -> Log all channels1/2
  Log all channels1/1 -> newPitchRes/1

== system dspcelpcoder/CELP Encoder/Frame Analysis/Classical LPC analysis/LPC Analysis/EmptySubsystem ==

== system dspcelpcoder/CELP Encoder/Frame Analysis/LSF Interpolation/LSF Interpolation/EmptySubsystem ==

== system dspcelpcoder/CELP Encoder/Frame Analysis/LSF Vector Quantization/LSF Split VQ/EmptySubsystem ==

== system dspcelpcoder/CELP Encoder/Frame Analysis/LSF Vector Quantization/LSF Split VQ./Split vector quantization of LSF ==
  EmptySubsystem : Subsystem  PropExecContextAcrossSSBoundary=on

== system dspcelpcoder/CELP Encoder/Frame Analysis/LSF Vector Quantization/Paliwal Weight  Computation/Calculation of Perceptual  Weighting Factors ==
  EmptySubsystem : Subsystem  PropExecContextAcrossSSBoundary=on

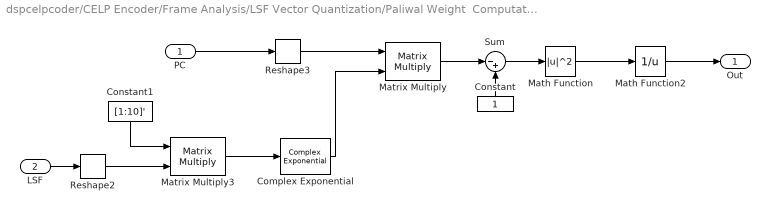
== system dspcelpcoder/CELP Encoder/Frame Analysis/LSF Vector Quantization/Paliwal Weight  Computation/LPCpowSpec ==
  PC : Inport  LatchInput=off
  LSF : Inport  Port=2  LatchInput=off
  Complex Exponential : dspmathops/Complex Exponential
  Constant : Constant  Orientation=up  VectorParams1D=off  SampleTime=-1
  Constant1 : Constant  Orientation=down  Value=[1:10]'  VectorParams1D=off  SampleTime=-1
  Math Function : Math  Operator=magnitude^2  SaturateOnIntegerOverflow=on
  Math Function2 : Math  Operator=reciprocal  SaturateOnIntegerOverflow=on
  Matrix Multiply : dspmtrx3/Matrix Multiply  numInputPorts=2  OptimizationLevel=None
  Matrix Multiply3 : dspmtrx3/Matrix Multiply  numInputPorts=2  OptimizationLevel=None
  Reshape2 : simulink/Math Operations/Reshape  OutputDimensionality=Row vector  OutputDimensions=[1,1]
  Reshape3 : simulink/Math Operations/Reshape  OutputDimensionality=Row vector  OutputDimensions=[1,1]
  Sum : Sum  Inputs=|-+  SaturateOnIntegerOverflow=on
  Out : Outport
  wires:
  Math Function2/1 -> Out/1
  Matrix Multiply/1 -> Sum/1
  PC/1 -> Reshape3/1
  Complex Exponential/1 -> Matrix Multiply/2
  Math Function/1 -> Math Function2/1
  Sum/1 -> Math Function/1
  Constant/1 -> Sum/2
  Reshape3/1 -> Matrix Multiply/1
  LSF/1 -> Reshape2/1
  Reshape2/1 -> Matrix Multiply3/2
  Constant1/1 -> Matrix Multiply3/1
  Matrix Multiply3/1 -> Complex Exponential/1

== system dspcelpcoder/CELP Encoder/Subframe Analysis/Innovation signal quantization/DocBlock/EmptySubsystem ==

== system dspcelpcoder/CELP Encoder/Subframe Analysis/Innovation signal quantization/Impulse Response/For Iterator Subsystem2 ==
  SigIn2 : Inport  LatchInput=off
  K : Inport  Port=2  LatchInput=off
  For Iterator : ForIterator  ResetStates=reset  IterationLimit=1  ShowIterationPort=off
  Time-Varying  Synthesis Filter 1/A(z). : dsparch4/Digital Filter  DialogController=dspDDGCreate  DialogControllerArgs=DataTag18  TypePopup=IIR (all poles)  IIRFiltStruct=Direct form II transposed  AllPoleFiltStruct=Lattice AR  FIRFiltStruct=Direct form  CoeffSource=Input port(s)  NumCoeffs=[1 -.95]  DenCoeffs=[1 0.1]  BiQuadCoeffs=[1 0.3 0.4 1 0.1 0.2]  LatticeCoeffs=[0.2 0.4]  denIgnore=off  FiltPerSampPopup=One filter per frame  IC=0  ICnum=0  ICden=0  roundingMode=Floor  overflowMode=off  ScaleValues=1  scaleValueFracLength=14  stageInFracLength=15  stageOutFracLength=15
  SigOut2 : Outport
  wires:
  K/1 -> Time-Varying  Synthesis Filter 1/A(z)./2
  SigIn2/1 -> Time-Varying  Synthesis Filter 1/A(z)./1
  Time-Varying  Synthesis Filter 1/A(z)./1 -> SigOut2/1

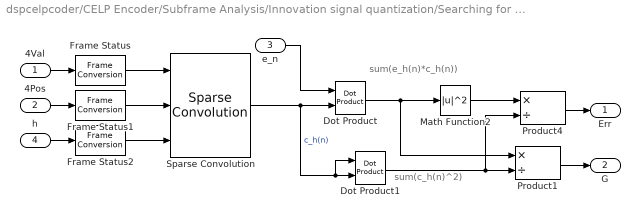
== system dspcelpcoder/CELP Encoder/Subframe Analysis/Innovation signal quantization/Searching for FCB pulse  positions and FCB gain/Computation of  Error and Gain ==
  note: sum(e_h(n)*c_h(n))
  note: sum(c_h(n)^2)
  4Val : Inport  LatchInput=off
  4Pos : Inport  Port=2  LatchInput=off
  e_n : Inport  Port=3  LatchInput=off
  h : Inport  Port=4  LatchInput=off
  Dot Product : simulink/Math Operations/Dot Product  OutDataType=sfix(16)  OutScaling=2^-10  DoSatur=on
  Dot Product1 : simulink/Math Operations/Dot Product  OutDataType=sfix(16)  OutScaling=2^-10  DoSatur=on
  Frame Status : FrameConversion
  Frame Status1 : FrameConversion
  Frame Status2 : FrameConversion
  Math Function2 : Math  Operator=magnitude^2  SaturateOnIntegerOverflow=on
  Product1 : Product  Inputs=*/  SaturateOnIntegerOverflow=on
  Product4 : Product  Inputs=*/  SaturateOnIntegerOverflow=on
  Sparse Convolution : dspcelplib/Sparse Convolution
  Err : Outport
  G : Outport  Port=2
  wires:
  Dot Product1/1 -> Product4/2, Product1/2
  Math Function2/1 -> Product4/1
  Dot Product/1 -> Math Function2/1, Product1/1
  Sparse Convolution/1 -> Dot Product/2, Dot Product1/2, Dot Product1/1  "c_h(n)"
  e_n/1 -> Dot Product/1
  4Val/1 -> Frame Status/1
  Product4/1 -> Err/1
  4Pos/1 -> Frame Status1/1
  h/1 -> Frame Status2/1
  Product1/1 -> G/1
  Frame Status/1 -> Sparse Convolution/1
  Frame Status1/1 -> Sparse Convolution/2
  Frame Status2/1 -> Sparse Convolution/3

== system dspcelpcoder/CELP Encoder/Subframe Analysis/Innovation signal quantization/Searching for FCB pulse  positions and FCB gain/Optimal Features ==
  SignBit : Inport  LatchInput=off
  Err : Inport  Port=2  LatchInput=off
  G : Inport  Port=3  LatchInput=off
  Pos : Inport  Port=4  LatchInput=off
  Data Type Conversion : DataTypeConversion  OutDataTypeMode=double  SaturateOnIntegerOverflow=on  RndMeth=Zero
  Data Type Conversion1 : DataTypeConversion  OutDataTypeMode=double  SaturateOnIntegerOverflow=on  RndMeth=Zero
  Delay1 : dspsigops/Delay  Orientation=left  dly_unit=Frames  delay=1  ic_detail=on  dif_ic_for_ch=off  dif_ic_for_dly=off  ic=0  reset_popup=None
  Feature  Concatenation : simulink/Math Operations/Matrix Concatenation  numInports=3  catMethod=Vertical
  Local maxima detector : Subsystem  PropExecContextAcrossSSBoundary=on
  Switch : Switch  Criteria=u2 ~= 0  InputSameDT=on
  Features : Outport
  wires:
  Local maxima detector/1(Flag) -> Switch/2
  Switch/1 -> Delay1/1, Features/1
  Delay1/1 -> Switch/3
  Feature  Concatenation/1 -> Switch/1
  Data Type Conversion/1 -> Feature  Concatenation/1
  Data Type Conversion1/1 -> Feature  Concatenation/2
  Pos/1 -> Data Type Conversion/1
  SignBit/1 -> Data Type Conversion1/1
  G/1 -> Feature  Concatenation/3
  Err/1 -> Local maxima detector/1(Err)

== system dspcelpcoder/CELP Encoder/Subframe Analysis/Innovation signal quantization/Searching for FCB pulse  positions and FCB gain/Partial decomposition of  Pitch Residual ==
  PitchRes : Inport  LatchInput=off
  Idx : Inport  Port=2  LatchInput=off
  Control : Inport  Port=3  LatchInput=off
  Data Type Conversion : DataTypeConversion  OutDataTypeMode=double  SaturateOnIntegerOverflow=on  RndMeth=Zero
  Data Type Conversion1 : DataTypeConversion  OutDataTypeMode=int32  SaturateOnIntegerOverflow=on  RndMeth=Zero
  "Select Rows I, I+1, ...,I+3" : dspcelplib/Select Rows  numRows=4
  Sort : dspstat3/Sort  DialogController=dspDDGCreate  DialogControllerArgs=DataTag20  otype=Value  dir=Ascending  sortAlg=Quick sort  roundingMode=Floor  overflowMode=off
  Variable Selector1 : dspindex/Variable Selector  rowsOrCols=Rows  IdxMode=Variable  Elements=[1 3]  ZerOneIdxMode=One-based  errmode=Generate Error
  4Val : Outport
  4Idx : Outport  Port=2
  wires:
  Data Type Conversion1/1 -> 4Idx/1
  Idx/1 -> "Select Rows I, I+1, ...,I+3"/1
  Data Type Conversion/1 -> Sort/1
  "Select Rows I, I+1, ...,I+3"/1 -> Data Type Conversion/1
  Sort/1 -> Data Type Conversion1/1, Variable Selector1/2
  PitchRes/1 -> Variable Selector1/1
  Variable Selector1/1 -> 4Val/1
  Control/1 -> "Select Rows I, I+1, ...,I+3"/2

== system dspcelpcoder/CELP Encoder/Subframe Analysis/Innovation signal quantization/Searching for FCB pulse  positions and FCB gain/Searching for FCB features ==
  EmptySubsystem : Subsystem  PropExecContextAcrossSSBoundary=on

== system dspcelpcoder/CELP Encoder/Subframe Analysis/Innovation signal quantization/Searching for FCB pulse  positions and FCB gain/Signal to sign bit ==
  Sig : Inport  LatchInput=off
  Constant : Constant  Value=+1  OutDataTypeMode=int32
  Constant1 : Constant  Value=-1  OutDataTypeMode=int32
  Switch : Switch
  SignBit : Outport
  wires:
  Sig/1 -> Switch/2
  Constant1/1 -> Switch/3
  Constant/1 -> Switch/1
  Switch/1 -> SignBit/1

== system dspcelpcoder/CELP Encoder/Subframe Analysis/Innovation signal quantization/filter/DocBlock ==
  EmptySubsystem : Subsystem  PropExecContextAcrossSSBoundary=on

== system dspcelpcoder/CELP Encoder/Subframe Analysis/Pitch Estimation/Open loop  Pitch estimation/Open Loop Pitch Estimation ==
  EmptySubsystem : Subsystem  PropExecContextAcrossSSBoundary=on

== system dspcelpcoder/CELP Encoder/Subframe Analysis/Pitch Estimation/Open loop  Pitch estimation/sum(r(n-D)^2) ==
  ACB : Inport  LatchInput=off
  Autocorrelation : dspstat3/Autocorrelation  DialogController=dspDDGCreate  DialogControllerArgs=DataTag26  AllPositiveLags=off  maxlag=0  bias=None  domain=Time  roundingMode=Floor  overflowMode=off
  Constant : Constant  Orientation=up  Value=eps  VectorParams1D=off  SampleTime=-1
  For Iterator : ForIterator  IterationLimit=128
  Log all channels : dspcelplib/Log all channels  outType=Column vector  numRow=128  numCol=4  dType=double
  "Select Rows D, D+1,...D+39" : dspcelplib/Select Rows  numRows=40
  Sum3 : Sum  Inputs=|++  SaturateOnIntegerOverflow=on
  sum(r(n-D)^2) : Outport
  wires:
  Sum3/1 -> Log all channels/1
  Autocorrelation/1 -> Sum3/1
  Constant/1 -> Sum3/2
  Log all channels/1 -> sum(r(n-D)^2)/1
  [E1] -> Log all channels/2
  For Iterator/1 -> [E1], "Select Rows D, D+1,...D+39"/2  "r(n-D)"
  ACB/1 -> "Select Rows D, D+1,...D+39"/1
  "Select Rows D, D+1,...D+39"/1 -> Autocorrelation/1  "r(n-D)"

== system dspcelpcoder/CELP Encoder/Subframe Analysis/Pitch Estimation/Pitch Estimation/EmptySubsystem ==

== system dspcelpcoder/CELP Encoder/Subframe Analysis/Pitch Residual computation/DocBlock/EmptySubsystem ==

== system dspcelpcoder/CELP Decoder/Subframe Synthesis/Reconstruction of  Speech Subframe/Harmonic Shaper/Energy normalization/Subsystem1 ==
  In1 : Inport  LatchInput=off
  Dot Product : simulink/Math Operations/Dot Product  OutDataType=sfix(16)  OutScaling=2^-10  DoSatur=on
  Out1 : Outport
  wires:
  In1/1 -> Dot Product/1, Dot Product/2
  Dot Product/1 -> Out1/1

== system dspcelpcoder/CELP Decoder/Subframe Synthesis/Reconstruction of  Speech Subframe/Harmonic Shaper/Energy normalization/Subsystem2 ==
  In1 : Inport  LatchInput=off
  Dot Product : simulink/Math Operations/Dot Product  OutDataType=sfix(16)  OutScaling=2^-10  DoSatur=on
  Out1 : Outport
  wires:
  Dot Product/1 -> Out1/1
  In1/1 -> Dot Product/2, Dot Product/1
